simulink model "Reference_CVS"  (R2026a)
settings: Solver=ode1  StopTime=40
InitFcn:
  | %motor_control_init_m
  | %clear all
  | %close all
  | %clc
  | b=1e-8
  | StepSize = 1e-4;
  | N=1e-17;
  | 
  | VLV_0 =0;%120; %120
  | VA_0 = 0;%300; %300
  | VRV_0 = 0;%130;
  | VP_0 = 0;%500;
  | VLA_0 = 0;%20;
  | VV_0=5000;
  | VRA_0=0;
  | 
  | 
  | QLV_0 = 0;
  | QLA_0 = 0;
  | QP_0 = 0;
  | 
  | bh = 0;
  | th =0;
  | 
  | X_0 = [VLV_0 VA_0 VV_0 VP_0  VLA_0  VRA_0 VRV_0];
  | 
  | 
  | V0 = 10;
  | 
  | K1=.0004;%0.0001
  | K2=0.0009;%0.0009
  | KA=1;%1
  | C1=0.000000003;%0.0000003
  | lambda=6000;%3000
  | X_00 = [VLV_0 VA_0 VV_0 VRV_0];
  | 
  | r2 = 0.05/2;
  | A2 = pi*r2^2;
  | h2 = 0.63;
  | V2 = A2*h2;
  | 
  | 
  | r3 = 0.05/2;
  | A3 = pi*r3^2;
  | h3 = 0.63;
  | V3 = A3*h3;
  | 
  | 
  | rho = 997;
  | gg = 9.81;
  | %
  | init_min=0;
  | init_max=0;
  | %
  | PWM_Period =  StepSize;
  | PWM_Period_g1 = PWM_Period;
  | PWM_Period_g2 =PWM_Period;
  | PWM_Period_g3 = PWM_Period;
  | PWM_Period_g4 = PWM_Period;
  | PWM_Period_g5 = PWM_Period;
  | PWM_Period_P2_escape = PWM_Period;
  | PWM_Period_P3_escape = PWM_Period;
  | filter_c=100;
  | dt = StepSize;
  | dt_k = dt;
  | rho_g=1.537408456055604
  | Pvac = 0;
  | P1refmmHg = 1600;
  | P2refmmHg = 30;
  | 
  | 
  | P2_ref_freq = 1;
  | P2_ref_bias = 50;
  | P2_ref_amp = 0;
  | P2_ref_shift = 0;
  | Kp = 1;
  | Ki =1;
  | Kd=1;
  | 
  | 
  | P3_ref_freq = 1;
  | P3_ref_bias = 30;
  | P3_ref_amp = 0;
  | P3_ref_shift = 0;
  | 
  | Q_Sys_std = 1;
  | R_Meas_std = 1;
  | kalmanP_in= [133.32*[100 1 10 10 1]]';
  | kalmanQ_in = [1e-3 1e-3]';
  | y_kalman_ini = [133.32*[100 1 10 10 1] 1e-3 1e-3 1e-3]';
  | P_kalman_ini = R_Meas_std^2*eye(8);
  | %P_kalman_ini = R_Meas_std^2*eye(8);
  | %P_kalman_in1 = R_Meas_std^2*eye(8);
  | 
  | 
  | w_gp_0 = 1e-3;
  | i_gp_0 = 1e-3;
  | w_vad_0 = 1e-3;
  | i_vad_0 = 1e-3;
  | 
  | 
  | 
  | 
  | 
  | % e_min = 0.075;
  | % %e_max = 3;
  | % e_max_ill = 1.5; PA_0 = 85;
  | % tau_RA = 1.8;  tau_RV = 3;% 2.3762;
  | % V_total = 5500; V0_la = 70; V0_lv = 120; V0 = 10;
  | % RA = 1.2; Ra = 0.0005;
  | % Rm = 0.0003; Rv = 0.005;
  | % R = [RA Ra Rm Rv];
  | % g = [1/RA 1/Ra 1/Rm 1/Rv];
  | %
  | % CA = tau_RA/RA; CV = tau_RV/Rv;
  | %
  | % V0_aortic = PA_0*CA;
  | % PLV_0 = (V0_lv - V0)*e_min;
  | % CLA = V0_la/PLV_0;
  | % C = [CA CV CLA];
  | % e = [1/CA 1/CV 1/CLA];
  | %
  | % V0_venous = V_total - (V0_aortic + V0_la + V0_lv);
  | % PLA_0 = PLV_0;
  | % PV_0 = V0_venous/CV;
  | 
  | 
  | 
  | 
  | 
  | 
  | 
  | 
  | % stepsize = 1e-4;
  | 
  | % SS=1;
  | 
  | 
  | 
  | 
  | 
  | %global RFa RFp
  | %RFa = 1;
  | %RFmv = 1;
  | 
  | 
  | 
  | 
  | 
  | %L_AV =  0.000232;
  | %L_mv =  0.0001;
  | %L_P =  0.000128;
  | a=0;
  | 
  | 
  | 
  | 
  | 
  | %L= [L_mv];
  | 
  | 
  | 
  | 
  | 
  | % gLV =42;%25;
  | % gA = 0.9225;%0.75;  %0.8;%0.725; %1.11;
  | % gV = 70;%10000;
  | % gRV =210;
  | % gP =5;%15 %10;
  | % gLA = 1000; %1000;
  | %
  | %
  | % G = [gLV gA gV gRV gP gLA];
  | %
  | %
  | % eA =0.5225;%0.725;%1; %0.925;%0.83; %0.65;%0.95;
  | % eV =0.002425;%0.00245;%0.00125;
  | % eP =0.1; %0.01%0.1;
  | % eLA =0.1025;%0.1105%0.1175;%0.15; % 0.15;
  | %
  | %
  | % E = [eA eV eP eLA];
  | %
  | %
  | % ZZ = 0.75;
  | % PP = 0.95;
  | %
  | % V_T = 5000;
  | % VLV_0 =105;%120; %120
  | % VA_0 = 160;%300; %300
  | % VRV_0 = 110;%130;
  | % VP_0 = 200;%500;
  | % VLA_0 = 105;%20;
  | % VV_0=0;
  | % QLV_0 = 0;
  | % QLA_0 = 0;
  | % QP_0 = 0;
  | %
  | % X_0 = [VLV_0 VA_0 VRV_0 VP_0 VLA_0];
  | % %BF_0 = [0 0 0];
  | %
  | %
  | % V0 = 10;
  | 
  | 
  | %Delay = 0.85;
  | 
  | 
  | 
  | 
  | 
  | %%CVS PARAMETERS NEW
  | 
  | 
  | stepsize = 1e-4;
  | 
  | 
  | SS=0.8;
libraries: powerlib_meascontrol x12, simulink x8, cstblocks x6
(part 1 of 2)
settings Model: Creator=ehd  LastModifiedBy=ehd

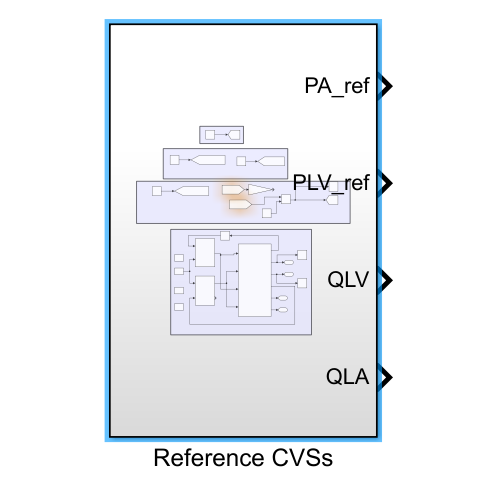
[thumbnail: Simulink's stored preview of the top-level diagram]
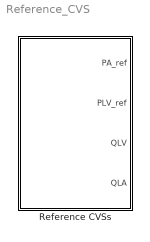
== system Reference_CVS ==
  Reference CVSs : Subsystem

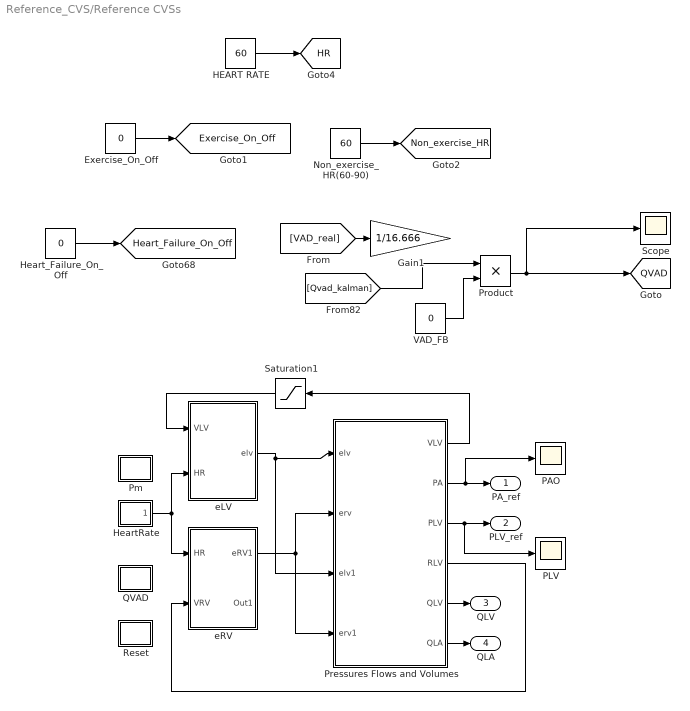
== system Reference_CVS/Reference CVSs ==
  Exercise_On_Off : Constant  Value=0
  Gain1 : Gain  Gain=1/16.666
  HEART RATE : Constant  Value=60
  HeartRate : Subsystem
  Heart_Failure_On_Off : Constant  Value=0
  Non_exercise_HR(60-90) : Constant  Value=60
  PAO : Scope
      settings: ActiveDisplayYMinimum=-0.039798343715390615  ActiveDisplayYMaximum=0.35818509343851557
  PLV : Scope
      settings: ActiveDisplayYMinimum=-23.924884385972419  ActiveDisplayYMaximum=6.1036636998176323  DataLoggingVariableName=ScopeData2
  Pm : Subsystem
  Pressures Flows and Volumes : Subsystem
  Product : Product
  QVAD : Subsystem
  Reset : Subsystem
  Saturation1 : Saturate  UpperLimit=500  LowerLimit=-100
  Scope : Scope
      settings: ActiveDisplayYMinimum=-1  ActiveDisplayYMaximum=1  DataLoggingVariableName=ScopeData3
  VAD_FB : Constant  Value=0
  eLV : Subsystem
  eRV : Subsystem
  PA_ref : Outport  VectorParamsAs1DForOutWhenUnconnected=off
  PLV_ref : Outport  Port=2  VectorParamsAs1DForOutWhenUnconnected=off
  QLV : Outport  Port=3  VectorParamsAs1DForOutWhenUnconnected=off
  QLA : Outport  Port=4  VectorParamsAs1DForOutWhenUnconnected=off
  tag scope: Exercise_On_Off=global, HR=global, Heart_Failure_On_Off=global, Non_exercise_HR=global, QVAD=global
  wires:
  Saturation1/1 -> eLV/1(VLV)
  [Qvad_kalman] -> Product/1
  [VAD_real] -> Gain1/1
  Pressures Flows and Volumes/5(QLV) -> QLV/1
  Pressures Flows and Volumes/6(QLA) -> QLA/1
  Pressures Flows and Volumes/2(PA) -> PA_ref/1, PAO/1
  Pressures Flows and Volumes/3(PLV) -> PLV_ref/1, PLV/1
  Pressures Flows and Volumes/1(VLV) -> Saturation1/1
  eLV/1(elv) -> Pressures Flows and Volumes/1(elv), Pressures Flows and Volumes/3(elv1)
  HeartRate/1(Out1) -> eLV/2(HR), eRV/1(HR)
  eRV/1(eRV1) -> Pressures Flows and Volumes/2(erv), Pressures Flows and Volumes/4(erv1)
  Pressures Flows and Volumes/4(RLV) -> eRV/2(VRV)
  VAD_FB/1 -> Product/2
  Product/1 -> [QVAD], Scope/1
  HEART RATE/1 -> [HR]
  Heart_Failure_On_Off/1 -> [Heart_Failure_On_Off]
  Non_exercise_HR(60-90)/1 -> [Non_exercise_HR]
  Exercise_On_Off/1 -> [Exercise_On_Off]

== system Reference_CVS/Reference CVSs/HeartRate ==
  Display : Display
  Display1 : Display
  Display2 : Display
  Switch2 : Switch  Criteria=u2 > Threshold  SaturateOnIntegerOverflow=off  InputSameDT=off
  Out1 : Outport
  tag scope: insan=global
  wires:
  Switch2/1 -> Display2/1, [insan]
  [Non_exercise_HR] -> Display1/1, Switch2/3
  [Exercise_On_Off] -> Switch2/2
  [HR] -> Display/1, Switch2/1, Out1/1

== system Reference_CVS/Reference CVSs/Pm ==
  note: y = -0,0333x 2 + 11,667x - 580
  note: y = -0,3333x2 + 116,67x - 5800R² = 1
  Add18 : Sum
  Add19 : Sum
  Constant20 : Constant  Value=-580
  Gain1 : Gain  Gain=1/100
  Gain2 : Gain  Gain=-0.0333
  Gain3 : Gain  Gain=11.667
  PID : Subsystem  Commented=on
  Product15 : Product
  Scope : Scope
      settings: ActiveDisplayYMinimum=3.007  ActiveDisplayYMaximum=5.007
  tag scope: PM=global
  wires:
  Gain1/1 -> Scope/1, [PM]
  Constant20/1 -> Add19/2
  Product15/1 -> Gain2/1
  Add18/1 -> Add19/1
  [HR] -> Gain3/1, Product15/2, Product15/1
  Gain3/1 -> Add18/2
  Gain2/1 -> Add18/1
  Add19/1 -> Gain1/1

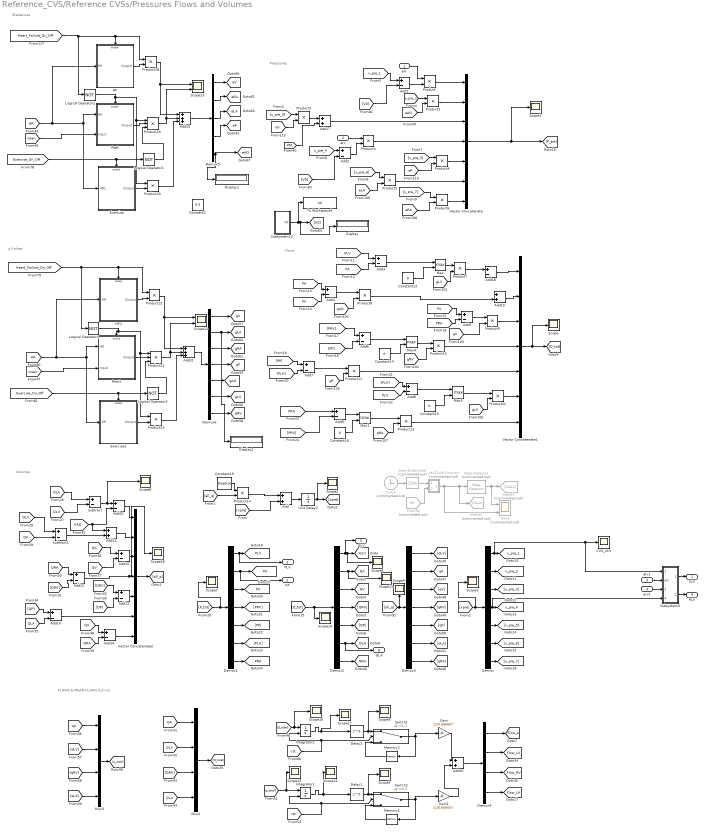
== system Reference_CVS/Reference CVSs/Pressures Flows and Volumes ==
  note: FLOWS & MEAN FLOWS (L/min)
  note: Elastances
  note: g Values
  note: Presssures
  note: Flows
  note: Volumes
  elv : Inport
  erv : Inport  Port=2
  elv1 : Inport  Port=3
  erv1 : Inport  Port=4
  Add{,11,17,19..20} (5 alike) : Sum
  Add{1..10,12..16,18} (16 alike) : Sum  Inputs=+-
  Add21 : Sum  Inputs=+++
  Add25 : Sum  Inputs=+++
  CVS_VLV : Scope
      settings: DataLoggingVariableName=ScopeData4
  Clock : Clock  Commented=on
      settings: Decimation=10000000
  Constant{13..16} (4 alike) : Constant  Value=0
  Constant19 : Constant  Value=stepsize
  Constant2 : Constant  Value=0.3
  Delay1 : Delay  DelayLength=5
  Delay2 : Delay  DelayLength=5
  Demux{,1..3,6} (5 alike) : Demux  Outputs=7
  Demux4 : Demux
  Demux5 : Demux  Outputs=5
  Display : Display
  Display1 : Display
  Display2 : Display
  Edge Detector : powerlib_meascontrol/Logic/Edge Detector  Commented=on  model=Falling  ic=0  Ts=0
      settings: SourceProductName=Simscape Electrical
  Exercise : Subsystem  TreatAsAtomicUnit=on
  Exercise2 : Subsystem  TreatAsAtomicUnit=on
  From90 : From  Commented=on  GotoTag=HR  TagVisibility=global
  Gain : Gain  Gain=1/16.666667
  Gain1 : Gain  Gain=1/16.666667
  Goto32 : Goto  Commented=on  GotoTag=Reset
  Goto55 : Goto  Commented=on  GotoTag=AAAA
  HF : Subsystem  TreatAsAtomicUnit=on
  HF1 : Subsystem  TreatAsAtomicUnit=on
  Integrator1 : Integrator  ExternalReset=either
  Integrator2 : Integrator  ExternalReset=either
  Logical Operator{1..4} (4 alike) : Logic  Operator=NOT  AllPortsSameDT=off  OutDataTypeStr=boolean
  MATLAB Function : MATLAB Function  Commented=on  TreatAsAtomicUnit=on
  Max{,1,4..5} (4 alike) : MinMax  Function=max  Inputs=2
  Memory1 : Memory  InheritSampleTime=on
  Memory2 : Memory  InheritSampleTime=on
  Mux2 : Mux
  Mux3 : Mux
  Product{,1..14,18,20..21,23} (19 alike) : Product
  Product19 : Product  Inputs=3
  Product22 : Product  Inputs=3
  Rest : Subsystem  TreatAsAtomicUnit=on
  Rest1 : Subsystem  TreatAsAtomicUnit=on
  Scope{,1..11,14..18} (17 alike) : Scope
      Scope settings: ActiveDisplayYMinimum=-77.48033  ActiveDisplayYMaximum=390.18057  DataLoggingVariableName=ScopeData3
      Scope1 settings: ActiveDisplayYMinimum=-17.90547  ActiveDisplayYMaximum=127.32097  DataLoggingVariableName=ScopeData4
      Scope10 settings: ActiveDisplayYMinimum=957.88839  ActiveDisplayYMaximum=957.93755  DataLoggingVariableName=ScopeData12
      Scope11 settings: ActiveDisplayYMinimum=-27.48687  ActiveDisplayYMaximum=51.0539  DataLoggingVariableName=ScopeData10
      Scope14 settings: ActiveDisplayYMinimum=-110.80263  ActiveDisplayYMaximum=77.31742
      Scope15 settings: ActiveDisplayYMinimum=-5789.58317  ActiveDisplayYMaximum=-2381.5007  DataLoggingVariableName=ScopeData2
      Scope16 settings: ActiveDisplayYMinimum=1027.76879  ActiveDisplayYMaximum=5015.29115  DataLoggingVariableName=ScopeData3
      Scope17 settings: ActiveDisplayYMinimum=-44.98014  ActiveDisplayYMaximum=404.82124  DataLoggingVariableName=ScopeData4
      Scope18 settings: ActiveDisplayYMinimum=2390.88881  ActiveDisplayYMaximum=2481.24108  DataLoggingVariableName=ScopeData5
      Scope2 settings: ActiveDisplayYMinimum=-34.04375  ActiveDisplayYMaximum=306.39376  DataLoggingVariableName=ScopeData3
      Scope3 settings: ActiveDisplayYMinimum=-92.27651  ActiveDisplayYMaximum=239.55796  DataLoggingVariableName=ScopeData3
      Scope4 settings: ActiveDisplayYMinimum=-3614.79854  ActiveDisplayYMaximum=3696.63533
      Scope5 settings: ActiveDisplayYMinimum=-10.26706  ActiveDisplayYMaximum=83.80402  DataLoggingVariableName=ScopeData2
      Scope6 settings: ActiveDisplayYMinimum=-1637.52208  ActiveDisplayYMaximum=5158.92158  DataLoggingVariableName=ScopeData9
      Scope7 settings: ActiveDisplayYMinimum=75.32296  ActiveDisplayYMaximum=84.1275  DataLoggingVariableName=ScopeData3
      Scope8 settings: ActiveDisplayYMinimum=-106.50454  ActiveDisplayYMaximum=958.54088  DataLoggingVariableName=ScopeData10
      Scope9 settings: ActiveDisplayYMinimum=-10.26706  ActiveDisplayYMaximum=83.80402  DataLoggingVariableName=ScopeData3
  Scope12 : Scope  NumInputPorts=2
      settings: ActiveDisplayYMinimum=-0.0275  ActiveDisplayYMaximum=0.2475  DataLoggingVariableName=ScopeData3
  Scope13 : Scope  NumInputPorts=2
      settings: ActiveDisplayYMinimum=-31.25  ActiveDisplayYMaximum=281.25  DataLoggingVariableName=ScopeData2
  Subsystem13 : Subsystem
  Subsystem5 : Subsystem
  Subtract : Sum  Inputs=+-
  Subtract1 : Sum  Inputs=+-
  Switch1 : Switch  Threshold=1  SaturateOnIntegerOverflow=off  InputSameDT=off
  Switch2 : Switch  Threshold=1  SaturateOnIntegerOverflow=off  InputSameDT=off
  To Workspace5 : ToWorkspace  VariableName=V0  SampleTime=-1
      settings: Save2DSignal=2-D array (concatenate along first dimension)
  Unit Delay2 : UnitDelay  InitialCondition=X_0  SampleTime=-1
  Vector Concatenate : Concatenate  NumInputs=7
  Vector Concatenate1 : Concatenate  NumInputs=7
  Vector Concatenate2 : Concatenate  NumInputs=7
  Wave : Scope  Commented=on  NumInputPorts=2
      settings: ActiveDisplayYMinimum=-0.125  ActiveDisplayYMaximum=1.125  DataLoggingVariableName=ScopeData2
  Zero-Order Hold : ZeroOrderHold  Commented=on  SampleTime=-1
  VLV : Outport
  PA : Outport  Port=2  VectorParamsAs1DForOutWhenUnconnected=off
  PLV : Outport  Port=3  VectorParamsAs1DForOutWhenUnconnected=off
  RLV : Outport  Port=4
  QLV : Outport  Port=5  VectorParamsAs1DForOutWhenUnconnected=off
  QLA : Outport  Port=6  VectorParamsAs1DForOutWhenUnconnected=off
  tag scope: Flow_A=global, Flow_LA=global, Flow_LV=global, Flow_RV=global, PA=global, PLV=global, PRA=global, PV=global, QA=global, QLA=global, QLV=global, QRA=global, QV=global, eAO=global, eLA=global, eP=global, eRA=global, eV=global, gAO=global, gLA=global, gLV=global, gP=global, gRA=global, gRV=global, gV=global, qA=global, x_pre_1=global, x_pre_2=global, x_pre_4=global
  wires:
  Product12/1 -> Vector Concatenate1/6
  [QRV] -> Mux2/3
  [QA] -> Mux2/1
  Mux2/1 -> [Q_total]
  Demux4/1 -> [Flow_A]
  [qLV] -> Mux3/2
  Mux3/1 -> [q_total]
  [qRV] -> Mux3/3
  [qA] -> Mux3/1
  [QLV] -> Mux2/2
  [qLA] -> Mux3/4
  Add20/1 -> Demux4/1
  Demux4/4 -> [Flow_LA]
  Switch1/1 -> Gain/1, Memory2/1
  [QLA] -> Mux2/4
  Gain1/1 -> Add20/2
  Integrator2/1 -> Delay2/1, Scope17/1
  Memory2/1 -> Switch1/3
  [q_total] -> Integrator1/1, Scope15/1
  Integrator1/1 -> Delay1/1, Scope14/1
  Demux4/2 -> [Flow_LV]
  Memory1/1 -> Switch2/3
  Demux4/3 -> [Flow_RV]
  Delay2/1 -> Switch1/1, Scope9/1
  [Q_total] -> Integrator2/1, Scope16/1
  Delay1/1 -> Scope5/1, Switch2/1
  Switch2/1 -> Memory1/1, Gain1/1
  [rst] -> Switch2/2, Integrator1/2
  Gain/1 -> Add20/1
  [rst] -> Integrator2/2, Switch1/2
  Demux2/2 -> [QA], Scope11/1
  Demux5/5 -> Display1/1, [eAO]
  Demux6/5 -> [gAO]
  Product1/1 -> Vector Concatenate/2
  [eAO] -> Product1/2
  [x_pre_2] -> Product1/1
  Subsystem13/1(V0) -> [V0], Display/1, To Workspace5/1
  [HR] -> Rest1/1(HR), Exercise2/1(HR), HF1/1(HR)
  Demux5/3 -> [eLA]
  [Exercise_On_Off] -> Exercise/Enable, Logical Operator1/1
  Product19/1 -> Add25/2, Scope13/2
  Product21/1 -> Scope12/1, Add21/1
  Logical Operator1/1 -> Product19/3
  Demux6/7 -> [gRV]
  Logical Operator2/1 -> Rest/Enable, Product19/1, Product20/1
  Rest/1(Output) -> Product19/2
  [Exercise_On_Off] -> Exercise2/Enable, Logical Operator3/1
  Add25/1 -> Demux5/1
  [HR] -> Rest/1(HR), Exercise/1(HR1), HF/1(HR)
  Demux6/6 -> [gLV]
  Add21/1 -> Demux6/1
  Logical Operator4/1 -> Product22/1, Product23/1, Rest1/Enable
  HF1/1(Output) -> Product21/2
  Demux6/2 -> [gLA], Display2/1
  Demux6/1 -> [gV]
  [Heart_Failure_On_Off] -> HF/Enable, Product18/1, Logical Operator2/1
  [insan] -> Rest/2(Input)
  Demux5/4 -> [eP]
  Demux6/4 -> [gP]
  Product22/1 -> Add21/2, Scope12/2
  Product18/1 -> Scope13/1, Add25/1
  Exercise/1(Output) -> Product20/2
  Product20/1 -> Add25/3
  Logical Operator3/1 -> Product22/3
  Product23/1 -> Add21/3
  [Heart_Failure_On_Off] -> Logical Operator4/1, Product21/1, HF1/Enable
  Exercise2/1(Output) -> Product23/2
  Demux5/1 -> [eV]
  Rest1/1(Output) -> Product22/2
  Demux6/3 -> [gRA]
  Demux5/2 -> [eRA]
  HF/1(Output) -> Product18/2
  [insan] -> Rest1/2(Input)
  Demux/1 -> [x_pre_1], CVS_VLV/1, Subsystem5/1(In1)
  elv1/1 -> Subsystem5/2(elv)
  erv1/1 -> Subsystem5/3(erv)
  Demux/4 -> [x_pre_4], Subsystem5/4(In4)
  Subsystem5/1(Out1) -> VLV/1
  Subsystem5/2(Output1) -> RLV/1
  [PM] -> Add17/2
  [VAD] -> Add10/2, Add11/1
  Demux2/4 -> [QRV]
  [all_q] -> Scope4/1, Demux3/1
  Demux/2 -> [x_pre_2]
  From90/1 -> MATLAB Function/2(HR)
  MATLAB Function/1(y) -> Goto32/1, Edge Detector/1, Wave/2
  Demux1/2 -> [PA], PA/1
  Add19/1 -> Vector Concatenate1/2
  Product8/1 -> Add19/2
  Add18/1 -> Vector Concatenate1/1
  Product7/1 -> Add18/1
  Add11/1 -> Vector Concatenate2/2
  Add10/1 -> Vector Concatenate2/1
  Subtract1/1 -> Add11/2
  Subtract/1 -> Add10/1, Scope6/1
  [eV] -> Product2/2
  [V0] -> Add2/2
  [V0] -> Add1/2
  [eP] -> Product4/2
  [eLA] -> Product5/2
  [eRA] -> Product6/2
  [gRA] -> Product13/2
  [gLA] -> Product12/2
  [gP] -> Product11/2
  [gRV] -> Product10/2
  [gV] -> Product9/2
  [gAO] -> Product8/2
  [gLV] -> Product7/2
  Edge Detector/1 -> Goto55/1, Wave/1
  Demux3/7 -> [qRA]
  Demux3/6 -> [qLA]
  Demux3/5 -> [qP]
  Demux3/4 -> [qRV]
  Demux3/3 -> [qV]
  Demux3/2 -> [qA]
  Demux3/1 -> [qLV]
  Zero-Order Hold/1 -> MATLAB Function/1(u)
  Clock/1 -> Zero-Order Hold/1
  [QLV] -> Subtract/2
  Product9/1 -> Vector Concatenate1/3
  [Q_tot] -> Demux2/1, Scope10/1
  Unit Delay2/1 -> [xpre], Scope2/1
  Add/1 -> Unit Delay2/1
  Constant19/1 -> Product14/1
  Add14/1 -> Vector Concatenate2/6
  Add13/1 -> Vector Concatenate2/5
  Add12/1 -> Vector Concatenate2/4, Scope18/1
  Add15/1 -> Vector Concatenate2/3
  [x_pre_7] -> Product6/1
  [x_pre_6] -> Product5/1
  [x_pre_5] -> Product4/1
  [x_pre_4] -> Add2/1
  [x_pre_3] -> Product2/1
  Constant13/1 -> Max/2
  Add3/1 -> Max/1
  Add6/1 -> Max4/1
  Add9/1 -> Max1/1
  Add8/1 -> Max5/1
  Add17/1 -> Vector Concatenate/3
  Product2/1 -> Add17/1
  [all_q] -> Product14/2
  Vector Concatenate2/1 -> [all_q]
  Vector Concatenate1/1 -> Scope/1, [Q_tot]
  Vector Concatenate/1 -> Scope1/1, [P_tot]
  [QRA] -> Add16/2
  [QV] -> Add16/1
  Add16/1 -> Vector Concatenate2/7
  [QV] -> Add15/2
  [QA] -> Add15/1
  [QLA] -> Add14/2
  [QP] -> Add14/1
  [QP] -> Add13/2
  [QRV] -> Add13/1
  [QRV] -> Add12/2
  [QRA] -> Add12/1
  [QA] -> Subtract1/2
  [QLV] -> Subtract1/1
  [QLA] -> Subtract/1
  Demux2/3 -> [QV]
  Demux2/6 -> [QLA], QLA/1
  Demux2/5 -> [QP]
  Demux2/7 -> [QRA]
  Demux2/1 -> [QLV], Scope8/1, QLV/1
  Product13/1 -> Vector Concatenate1/7
  Max1/1 -> Product13/1
  Constant16/1 -> Max1/2
  [PRV] -> Add9/2
  [PRA] -> Add9/1
  Max5/1 -> Product12/1
  Constant15/1 -> Max5/2
  [PLV] -> Add8/2
  [PLA] -> Add8/1
  Product11/1 -> Vector Concatenate1/5
  Add7/1 -> Product11/1
  [PLA] -> Add7/2
  [PP] -> Add7/1
  Product10/1 -> Vector Concatenate1/4
  Max4/1 -> Product10/1
  [PP] -> Add6/2
  [PRV] -> Add6/1
  Constant14/1 -> Max4/2
  Add5/1 -> Product9/1
  [PRA] -> Add5/2
  [PV] -> Add5/1
  Add4/1 -> Product8/1
  [PV] -> Add4/2
  [PA] -> Add4/1
  Max/1 -> Product7/1
  [PA] -> Add3/2
  [PLV] -> Add3/1
  Demux1/3 -> [PV]
  Demux1/4 -> [PRV]
  Demux1/5 -> [PP]
  Demux1/6 -> [PLA]
  Demux1/7 -> [PRA]
  Demux1/1 -> [PLV], PLV/1
  [P_tot] -> Demux1/1, Scope7/1
  Product6/1 -> Vector Concatenate/7
  Product5/1 -> Vector Concatenate/6
  Product4/1 -> Vector Concatenate/5
  erv/1 -> Product3/1
  Product3/1 -> Vector Concatenate/4
  Add2/1 -> Product3/2
  Product/1 -> Vector Concatenate/1
  Add1/1 -> Product/2
  [x_pre_1] -> Add1/1
  Demux/7 -> [x_pre_7]
  Demux/6 -> [x_pre_6]
  Demux/5 -> [x_pre_5]
  Demux/3 -> [x_pre_3]
  [xpre] -> Demux/1, Scope3/1
  elv/1 -> Product/1
  [xpre] -> Add/2
  Product14/1 -> Add/1

== system Reference_CVS/Reference CVSs/QVAD ==
  Gain3 : Gain  Gain=16.666
  Product : Product
  Saturation : Saturate  UpperLimit=inf  LowerLimit=30
  Sine Wave : Sin  Amplitude=0.8  Frequency=0.4  SampleTime=0
  tag scope: VAD=global, VADQ=global
  wires:
  [QVAD] -> Gain3/1, [VADQ]
  Product/1 -> Saturation/1
  Sine Wave/1 -> Product/2
  Gain3/1 -> Product/1, [VAD]

== system Reference_CVS/Reference CVSs/Reset ==
  Clock2 : Clock
  Constant10 : Constant
  Constant11 : Constant  Value=0
  Constant12 : Constant  Value=10
  Mod2 : Math  Operator=mod  SignedPower=on
  Scope5 : Scope
      settings: ActiveDisplayYMinimum=-0.125  ActiveDisplayYMaximum=1.125  DataLoggingVariableName=ScopeData4
  Switch2 : Switch  Threshold=10-000001  SaturateOnIntegerOverflow=off  InputSameDT=off
  tag scope: dedect=global, rst=global
  wires:
  Clock2/1 -> Mod2/1
  Constant12/1 -> Mod2/2
  Constant10/1 -> Switch2/1
  Switch2/1 -> [rst], Scope5/1
  Constant11/1 -> Switch2/3
  Mod2/1 -> [dedect], Switch2/2

== system Reference_CVS/Reference CVSs/eLV ==
  VLV : Inport
  HR : Inport  Port=2
  Clock1 : Clock
  Constant : Constant  Value=3
  Display : Display
  LV_e_min : Subsystem
  Scope : Scope
      settings: ActiveDisplayYMinimum=-0.72024  ActiveDisplayYMaximum=3.41705
  Subsystem1 : Subsystem
  Switch : Switch  Criteria=u2 > Threshold  Threshold=0.9  SaturateOnIntegerOverflow=off  InputSameDT=off
  Switch1 : Switch  Criteria=u2 > Threshold  Threshold=0.9  SaturateOnIntegerOverflow=off  InputSameDT=off
  eLV1 : Subsystem
  eLVsick : Subsystem
  elv : Outport
  tag scope: eLV=global
  wires:
  eLVsick/1(Output) -> Switch/1
  Switch/1 -> Subsystem1/1(eLV_max), Display/1
  eLV1/1(Output) -> Switch1/1
  [Exercise_On_Off] -> Switch1/2
  Constant/1 -> Switch1/3
  Switch1/1 -> Switch/3
  [Heart_Failure_On_Off] -> Switch/2
  LV_e_min/1(eLV_min_O) -> Subsystem1/2(eLV_min)
  HR/1 -> Subsystem1/3(HR)
  VLV/1 -> LV_e_min/1(VLV)
  Subsystem1/1(elv) -> elv/1, [eLV], Scope/1
  Clock1/1 -> Subsystem1/4(t)

== system Reference_CVS/Reference CVSs/eRV ==
  HR : Inport
  VRV : Inport  Port=2
  Clock2 : Clock
  Display : Display
  RV_e_min : Subsystem
  Subsystem2 : Subsystem
  Switch : Switch  Criteria=u2 > Threshold  Threshold=0.9  SaturateOnIntegerOverflow=off  InputSameDT=off
  eRV2 : Subsystem
  eRVhf : Subsystem
  eRV1 : Outport
  Out1 : Outport  Port=2
  tag scope: eRV=global
  wires:
  Switch/1 -> Subsystem2/1(eRV_max), Display/1
  [Heart_Failure_On_Off] -> Switch/2
  eRVhf/1(Output) -> Switch/1
  eRV2/1(Output) -> Switch/3
  RV_e_min/1(eRV_min_O) -> Subsystem2/2(eRV_min)
  Subsystem2/1(eRV) -> eRV1/1, [eRV], Out1/1
  VRV/1 -> RV_e_min/1(VRV)
  HR/1 -> Subsystem2/4(HR)
  Clock2/1 -> Subsystem2/3(t)

== system Reference_CVS/Reference CVSs/Pm/PID ==
  s : Inport
  LTI System : cstblocks/LTI System  sys=tfa  IC=[]
  PID Controller : simulink/Continuous/PID Controller  Controller=PID  Form=Parallel  TimeDomain=Continuous-time  SampleTime=-1  IntegratorMethod=Forward Euler  FilterMethod=Forward Euler  ControllerParametersSource=internal  P=0  I=0.336541519886425  D=0  UseFilter=on  N=100  TunerSelectOption=Transfer Function Based (PID Tuner App)  InitialConditionSource=internal  InitialConditionForIntegrator=0  InitialConditionForFilter=0  DifferentiatorICPrevScaledInput=0  ExternalReset=none  TrackingMode=off  Kt=1  LimitOutput=off  UpperSaturationLimit=inf  LowerSaturationLimit=-inf  LinearizeAsGain=on  AntiWindupMode=none  Kb=1  POutMin=[]  POutMax=[]  IOutMin=[]  IOutMax=[]  DOutMin=[]  DOutMax=[]  NOutMin=[]  NOutMax=[]  SumOutMin=[]  SumOutMax=[]  SaturationOutMin=[]  SaturationOutMax=[]  PParamMin=[]  PParamMax=[]  IParamMin=[]  IParamMax=[]  DParamMin=[]  DParamMax=[]  NParamMin=[]  NParamMax=[]  KbParamMin=[]  KbParamMax=[]  KtParamMin=[]  KtParamMax=[]  KbOutMin=[]  KbOutMax=[]  KtOutMin=[]  KtOutMax=[]  IntegratorOutMin=[]  IntegratorOutMax=[]  FilterOutMin=[]  FilterOutMax=[]  SumI1OutMin=[]  SumI1OutMax=[]  SumI2OutMin=[]  SumI2OutMax=[]  SumI3OutMin=[]  SumI3OutMax=[]  SumI4OutMin=[]  SumI4OutMax=[]  SumDOutMin=[]  SumDOutMax=[]  DifferentiatorOutMin=[]  DifferentiatorOutMax=[]  FilterDiffOutCoefMin=[]  FilterDiffOutCoefMax=[]  ReciprocalOutMin=[]  ReciprocalOutMax=[]  SumDenOutMin=[]  SumDenOutMax=[]  SumNumOutMin=[]  SumNumOutMax=[]  DivideOutMin=[]  DivideOutMax=[]  IntegratorContinuousStateAttributes=''  IntegratorStateMustResolveToSignalObject=off  IntegratorRTWStateStorageClass=Auto  FilterContinuousStateAttributes=''  FilterStateMustResolveToSignalObject=off  FilterRTWStateStorageClass=Auto  ParallelPVariant=InternalParameters  IdealPVariant=Disabled  IVariant=InternalParameters  DVariant=InternalParameters  IntegratorVariant=Continuous  SatVariant=Disabled  AWVariant=Passthrough  PCopyVariant=Disabled  TRVariant=Disabled  FdbkBlocksVariant=Forward  IdealPFdbkVariant=Disabled  SatFdbkVariant=Disabled  DerivativeFilterVariant=ContFilter  NVariant=InternalParameters  NCopyVariant=Disabled  FilterICVariant=InternalICsFilter  IntegratorICVariant=InternalICs  ExternalResetVariant=Disabled  TRSumVariant=Passthrough  SumFdbkVariant=Disabled  SumVariant=Sum_PID
  Sum1 : Sum  Inputs=|+-
  To Workspace : ToWorkspace  VariableName=input  SampleTime=-1
  To Workspace1 : ToWorkspace  VariableName=output  SampleTime=-1
  E : Outport  VectorParamsAs1DForOutWhenUnconnected=off
  wires:
  PID Controller/1 -> To Workspace/1, LTI System/1
  s/1 -> Sum1/1
  Sum1/1 -> PID Controller/1
  LTI System/1 -> Sum1/2, E/1, To Workspace1/1

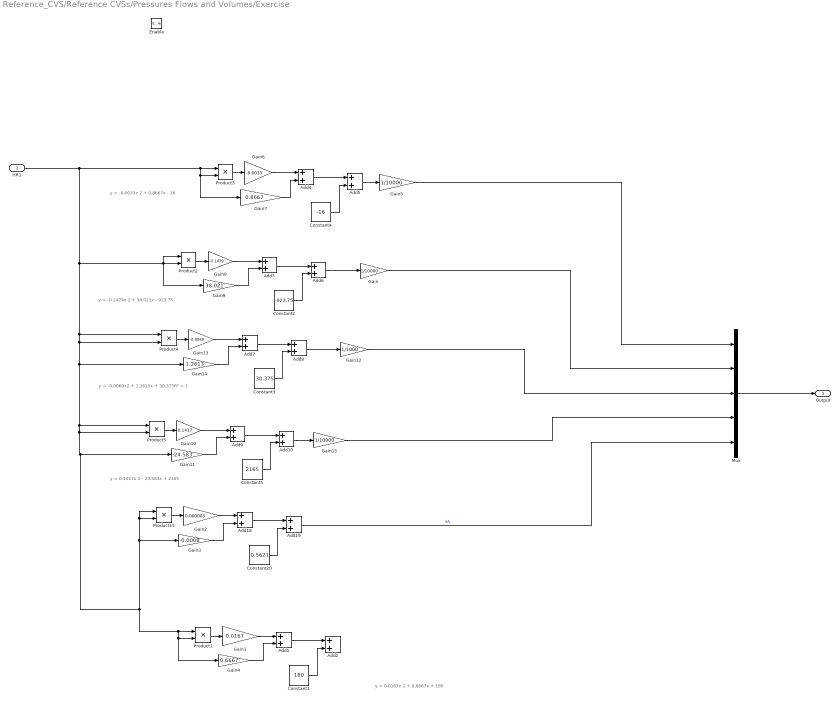
== system Reference_CVS/Reference CVSs/Pressures Flows and Volumes/Exercise ==
  note: y = -0,0033x 2 + 0,8667x - 16
  note: y = 0,1417x 2 - 24,583x + 2165
  note: y = -0,1479x 2 + 38,021x - 923,75
  note: y = -0,0069x2 + 1,2813x + 30,375R² = 1
  note: y = 0,0167x 2 + 0,6667x + 180
  HR1 : Inport
  Enable : EnablePort
  Add{1..10,18..19} (12 alike) : Sum
  Constant1 : Constant  Value=180
  Constant2 : Constant  Value=-923.75
  Constant20 : Constant  Value=0.5621
  Constant3 : Constant  Value=30.375
  Constant4 : Constant  Value=-16
  Constant5 : Constant  Value=2165
  Gain : Gain  Gain=1/10000
  Gain1 : Gain  Gain=0.0167
  Gain10 : Gain  Gain=0.1417
  Gain11 : Gain  Gain=-24.583
  Gain12 : Gain  Gain=1/1000
  Gain13 : Gain  Gain=-0.0069
  Gain14 : Gain  Gain=1.2813
  Gain15 : Gain  Gain=1/10000
  Gain2 : Gain  Gain=0.000003
  Gain3 : Gain  Gain=-0.0008
  Gain4 : Gain  Gain=0.6667
  Gain5 : Gain  Gain=1/10000
  Gain6 : Gain  Gain=-0.0033
  Gain7 : Gain  Gain=0.8667
  Gain8 : Gain  Gain=-0.1479
  Gain9 : Gain  Gain=38.021
  Mux : Mux  Inputs=5
  Product{1..5,15} (6 alike) : Product
  Output : Outport
  wires:
  Gain15/1 -> Mux/4
  Gain/1 -> Mux/2
  Product5/1 -> Gain10/1
  Gain7/1 -> Add4/2
  Gain14/1 -> Add7/2
  Product3/1 -> Gain6/1
  Gain5/1 -> Mux/1
  Add7/1 -> Add8/1
  Product2/1 -> Gain8/1
  Add5/1 -> Gain5/1
  Add6/1 -> Gain/1
  Constant2/1 -> Add6/2
  Gain6/1 -> Add4/1
  Add4/1 -> Add5/1
  Constant4/1 -> Add5/2
  Gain13/1 -> Add7/1
  Constant3/1 -> Add8/2
  Add10/1 -> Gain15/1
  Gain12/1 -> Mux/3
  Add8/1 -> Gain12/1
  Product4/1 -> Gain13/1
  Gain8/1 -> Add3/1
  Gain9/1 -> Add3/2
  Add3/1 -> Add6/1
  Add9/1 -> Add10/1
  Gain11/1 -> Add9/2
  Constant5/1 -> Add10/2
  Gain10/1 -> Add9/1
  Mux/1 -> Output/1
  Gain4/1 -> Add1/2
  Gain1/1 -> Add1/1
  Product1/1 -> Gain1/1
  Add1/1 -> Add2/1
  HR1/1 -> Product3/1, Product3/2, Gain7/1, Gain11/1, Product1/1, Product1/2, Gain4/1, Gain3/1, Product15/2, Product15/1, Product5/2, Product5/1, Gain14/1, Product4/2, Product4/1, Product2/2, Gain9/1, Product2/1
  Constant1/1 -> Add2/2
  Gain2/1 -> Add18/1
  Gain3/1 -> Add18/2
  Add18/1 -> Add19/1
  Constant20/1 -> Add19/2
  Product15/1 -> Gain2/1
  Add19/1 -> Mux/5  "eA"

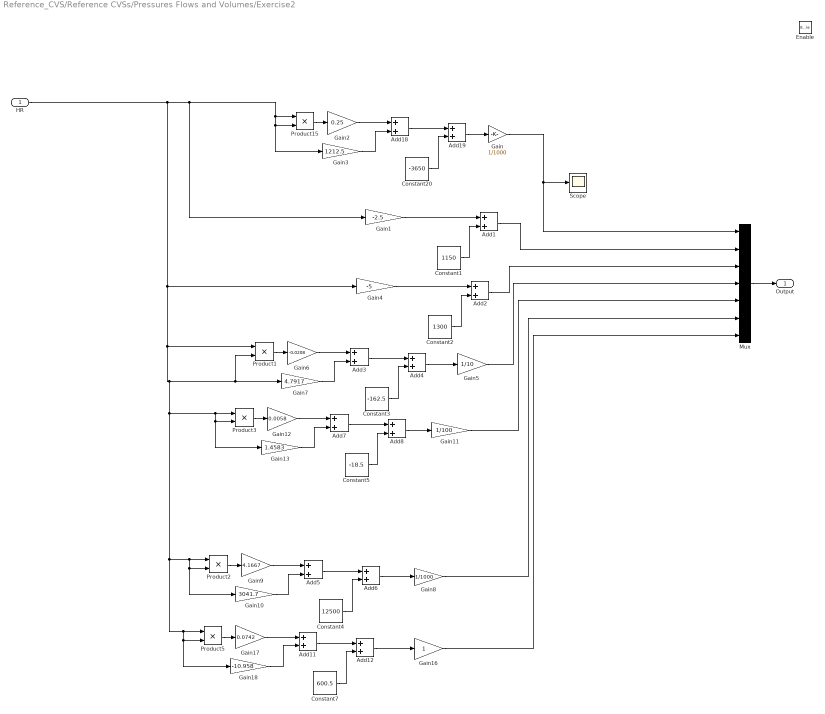
== system Reference_CVS/Reference CVSs/Pressures Flows and Volumes/Exercise2 ==
  HR : Inport
  Enable : EnablePort
  Add{1..8,11..12,18..19} (12 alike) : Sum
  Constant1 : Constant  Value=1150
  Constant2 : Constant  Value=1300
  Constant20 : Constant  Value=-3650
  Constant3 : Constant  Value=-162.5
  Constant4 : Constant  Value=12500
  Constant5 : Constant  Value=-18.5
  Constant7 : Constant  Value=600.5
  Gain : Gain  Gain=1/1000
  Gain1 : Gain  Gain=-2.5
  Gain10 : Gain  Gain=3041.7
  Gain11 : Gain  Gain=1/100
  Gain12 : Gain  Gain=0.0058
  Gain13 : Gain  Gain=1.4583
  Gain16 : Gain
  Gain17 : Gain  Gain=0.0742
  Gain18 : Gain  Gain=-10.958
  Gain2 : Gain  Gain=0.25
  Gain3 : Gain  Gain=1212.5
  Gain4 : Gain  Gain=-5
  Gain5 : Gain  Gain=1/10
  Gain6 : Gain  Gain=-0.0208
  Gain7 : Gain  Gain=4.7917
  Gain8 : Gain  Gain=1/1000
  Gain9 : Gain  Gain=4.1667
  Mux : Mux  Inputs=7
  Product{1..3,5,15} (5 alike) : Product
  Scope : Scope
      settings: ActiveDisplayYMinimum=60  ActiveDisplayYMaximum=80  DataLoggingVariableName=ScopeData9
  Output : Outport
  wires:
  Gain18/1 -> Add11/2
  Gain16/1 -> Mux/7
  Gain17/1 -> Add11/1
  HR/1 -> Gain4/1, Product1/1, Product3/1, Product3/2, Gain13/1, Gain18/1, Product5/2, Product5/1, Product2/1, Product2/2, Gain10/1, Product1/2, Gain7/1, Gain1/1, Product15/1, Product15/2, Gain3/1
  Add12/1 -> Gain16/1
  Constant7/1 -> Add12/2
  Add11/1 -> Add12/1
  Product5/1 -> Gain17/1
  Gain13/1 -> Add7/2
  Gain11/1 -> Mux/5
  Add8/1 -> Gain11/1
  Product3/1 -> Gain12/1
  Constant5/1 -> Add8/2
  Add7/1 -> Add8/1
  Gain12/1 -> Add7/1
  Mux/1 -> Output/1
  Gain2/1 -> Add18/1
  Gain/1 -> Mux/1, Scope/1
  Constant20/1 -> Add19/2
  Product15/1 -> Gain2/1
  Gain3/1 -> Add18/2
  Add19/1 -> Gain/1
  Add18/1 -> Add19/1
  Add1/1 -> Mux/2
  Constant1/1 -> Add1/2
  Gain1/1 -> Add1/1
  Gain4/1 -> Add2/1
  Add2/1 -> Mux/3
  Constant2/1 -> Add2/2
  Constant3/1 -> Add4/2
  Gain7/1 -> Add3/2
  Gain5/1 -> Mux/4
  Product1/1 -> Gain6/1
  Gain6/1 -> Add3/1
  Add4/1 -> Gain5/1
  Add3/1 -> Add4/1
  Add6/1 -> Gain8/1
  Constant4/1 -> Add6/2
  Gain10/1 -> Add5/2
  Gain8/1 -> Mux/6
  Add5/1 -> Add6/1
  Product2/1 -> Gain9/1
  Gain9/1 -> Add5/1

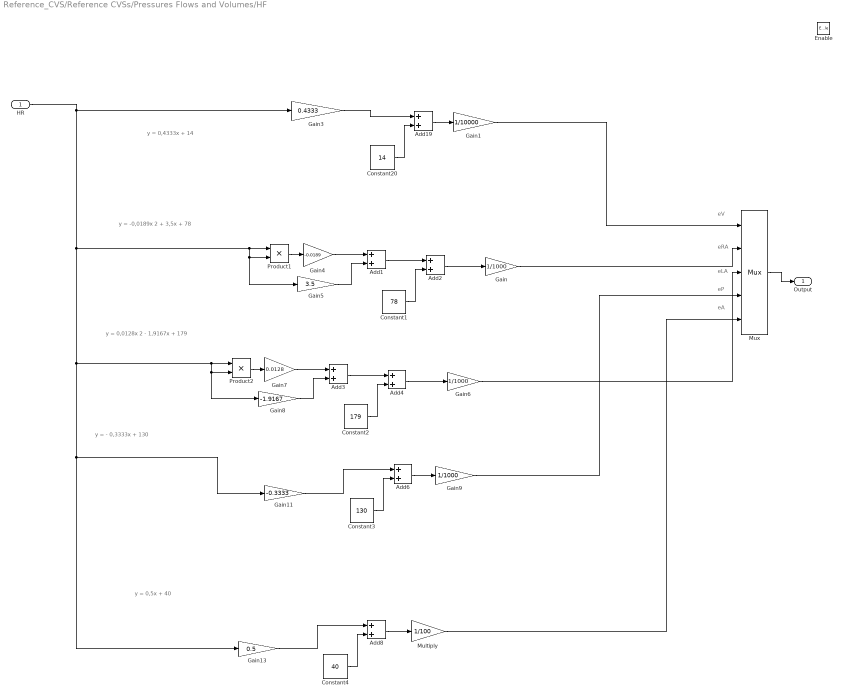
== system Reference_CVS/Reference CVSs/Pressures Flows and Volumes/HF ==
  note: eA
  note: eP
  note: eLA
  note: eRA
  note: eV
  note: y = 0,4333x + 14
  note: y = -0,0189x 2 + 3,5x + 78
  note: y = 0,0128x 2 - 1,9167x + 179
  note: y = - 0,3333x + 130
  note: y = 0,5x + 40
  HR : Inport
  Enable : EnablePort
  Add{1..4,6,8,19} (7 alike) : Sum
  Constant1 : Constant  Value=78
  Constant2 : Constant  Value=179
  Constant20 : Constant  Value=14
  Constant3 : Constant  Value=130
  Constant4 : Constant  Value=40
  Gain : Gain  Gain=1/1000
  Gain1 : Gain  Gain=1/10000
  Gain11 : Gain  Gain=-0.3333
  Gain13 : Gain  Gain=0.5
  Gain3 : Gain  Gain=0.4333
  Gain4 : Gain  Gain=-0.0189
  Gain5 : Gain  Gain=3.5
  Gain6 : Gain  Gain=1/1000
  Gain7 : Gain  Gain=0.0128
  Gain8 : Gain  Gain=-1.9167
  Gain9 : Gain  Gain=1/1000
  Multiply : Gain  Gain=1/100
  Mux : Mux  Inputs=5
  Product1 : Product
  Product2 : Product
  Output : Outport
  wires:
  HR/1 -> Gain3/1, Gain8/1, Product2/2, Product2/1, Gain11/1, Gain13/1, Gain5/1, Product1/2, Product1/1
  Gain13/1 -> Add8/1
  Constant4/1 -> Add8/2
  Add8/1 -> Multiply/1
  Multiply/1 -> Mux/5
  Mux/1 -> Output/1
  Gain9/1 -> Mux/4
  Constant3/1 -> Add6/2
  Gain11/1 -> Add6/1
  Add6/1 -> Gain9/1
  Gain6/1 -> Mux/3
  Product2/1 -> Gain7/1
  Constant2/1 -> Add4/2
  Add4/1 -> Gain6/1
  Gain8/1 -> Add3/2
  Gain7/1 -> Add3/1
  Add3/1 -> Add4/1
  Constant1/1 -> Add2/2
  Gain5/1 -> Add1/2
  Add2/1 -> Gain/1
  Gain4/1 -> Add1/1
  Product1/1 -> Gain4/1
  Gain/1 -> Mux/2
  Add1/1 -> Add2/1
  Add19/1 -> Gain1/1
  Gain1/1 -> Mux/1
  Constant20/1 -> Add19/2
  Gain3/1 -> Add19/1

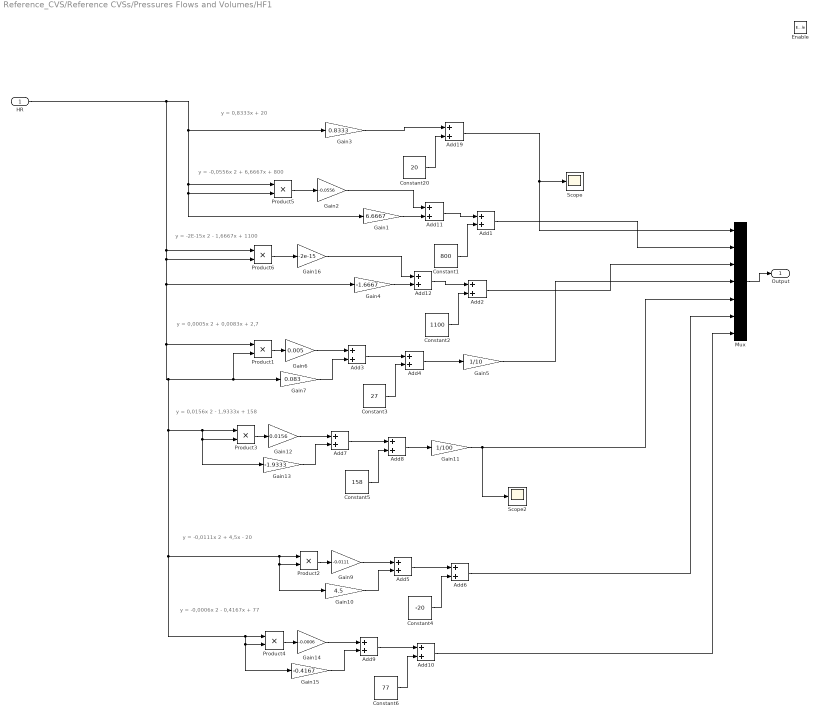
== system Reference_CVS/Reference CVSs/Pressures Flows and Volumes/HF1 ==
  note: y = -0,0006x 2 - 0,4167x + 77
  note: y = 0,0156x 2 - 1,9333x + 158
  note: y = -0,0556x 2 + 6,6667x + 800
  note: y = 0,0005x 2 + 0,0083x + 2,7
  note: y = 0,8333x + 20
  note: y = -2E-15x 2 - 1,6667x + 1100
  note: y = -0,0111x 2 + 4,5x - 20
  HR : Inport
  Enable : EnablePort
  Add{1..12,19} (13 alike) : Sum
  Constant1 : Constant  Value=800
  Constant2 : Constant  Value=1100
  Constant20 : Constant  Value=20
  Constant3 : Constant  Value=27
  Constant4 : Constant  Value=-20
  Constant5 : Constant  Value=158
  Constant6 : Constant  Value=77
  Gain1 : Gain  Gain=6.6667
  Gain10 : Gain  Gain=4.5
  Gain11 : Gain  Gain=1/100
  Gain12 : Gain  Gain=0.0156
  Gain13 : Gain  Gain=-1.9333
  Gain14 : Gain  Gain=-0.0006
  Gain15 : Gain  Gain=-0.4167
  Gain16 : Gain  Gain=-2e-15
  Gain2 : Gain  Gain=-0.0556
  Gain3 : Gain  Gain=0.8333
  Gain4 : Gain  Gain=-1.6667
  Gain5 : Gain  Gain=1/10
  Gain6 : Gain  Gain=0.005
  Gain7 : Gain  Gain=0.083
  Gain9 : Gain  Gain=-0.0111
  Mux : Mux  Inputs=7
  Product{1..6} (6 alike) : Product
  Scope : Scope
      settings: ActiveDisplayYMinimum=60  ActiveDisplayYMaximum=80  DataLoggingVariableName=ScopeData4
  Scope2 : Scope
      settings: ActiveDisplayYMinimum=0.88246  ActiveDisplayYMaximum=1.08246  DataLoggingVariableName=ScopeData5
  Output : Outport
  wires:
  HR/1 -> Gain3/1, Product5/2, Gain1/1, Product5/1, Gain7/1, Product1/2, Gain10/1, Product2/2, Product2/1, Product4/1, Product4/2, Gain15/1, Product3/1, Product3/2, Gain13/1, Product1/1, Gain4/1, Product6/2, Product6/1
  Add12/1 -> Add2/1
  Add5/1 -> Add6/1
  Gain2/1 -> Add11/1
  Constant20/1 -> Add19/2
  Gain4/1 -> Add12/2
  Add1/1 -> Mux/2
  Add3/1 -> Add4/1
  Add11/1 -> Add1/1
  Add10/1 -> Mux/7
  Gain5/1 -> Mux/4
  Constant5/1 -> Add8/2
  Add19/1 -> Scope/1, Mux/1
  Gain3/1 -> Add19/1
  Gain15/1 -> Add9/2
  Add9/1 -> Add10/1
  Gain14/1 -> Add9/1
  Product3/1 -> Gain12/1
  Constant1/1 -> Add1/2
  Mux/1 -> Output/1
  Constant2/1 -> Add2/2
  Gain6/1 -> Add3/1
  Constant4/1 -> Add6/2
  Product2/1 -> Gain9/1
  Add7/1 -> Add8/1
  Gain7/1 -> Add3/2
  Add8/1 -> Gain11/1
  Product1/1 -> Gain6/1
  Gain11/1 -> Scope2/1, Mux/5
  Gain9/1 -> Add5/1
  Gain10/1 -> Add5/2
  Constant3/1 -> Add4/2
  Add2/1 -> Mux/3
  Gain16/1 -> Add12/1
  Gain12/1 -> Add7/1
  Constant6/1 -> Add10/2
  Gain13/1 -> Add7/2
  Product4/1 -> Gain14/1
  Add4/1 -> Gain5/1
  Gain1/1 -> Add11/2
  Product5/1 -> Gain2/1
  Product6/1 -> Gain16/1
  Add6/1 -> Mux/6

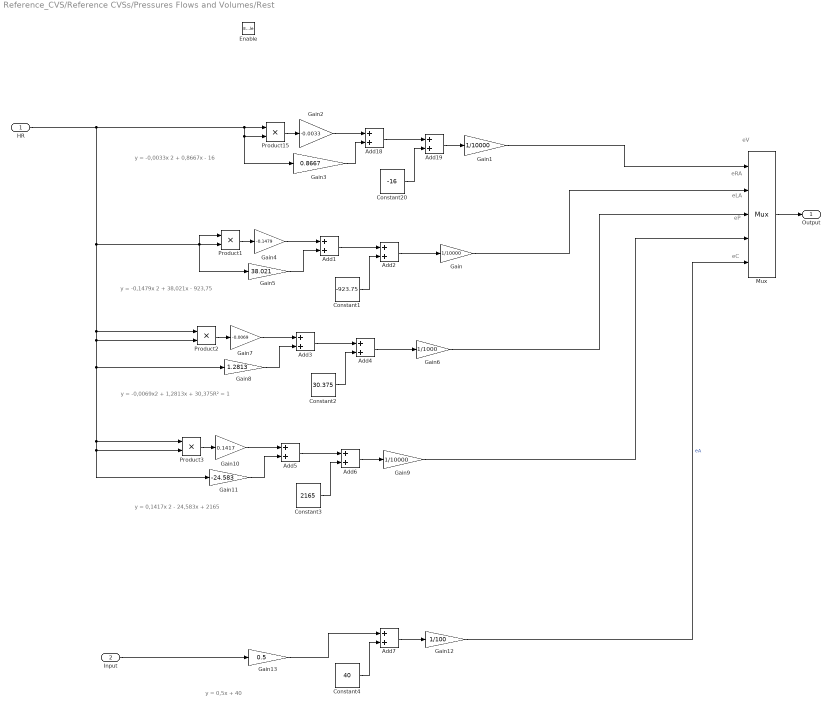
== system Reference_CVS/Reference CVSs/Pressures Flows and Volumes/Rest ==
  note: eV
  note: y = 0,5x + 40
  note: y = -0,1479x 2 + 38,021x - 923,75
  note: y = -0,0069x2 + 1,2813x + 30,375R² = 1
  note: y = 0,1417x 2 - 24,583x + 2165
  note: eP
  note: eLA
  note: eRA
  note: y = -0,0033x 2 + 0,8667x - 16
  note: eC
  HR : Inport
  Input : Inport  Port=2
  Enable : EnablePort
  Add{1..7,18..19} (9 alike) : Sum
  Constant1 : Constant  Value=-923.75
  Constant2 : Constant  Value=30.375
  Constant20 : Constant  Value=-16
  Constant3 : Constant  Value=2165
  Constant4 : Constant  Value=40
  Gain : Gain  Gain=1/10000
  Gain1 : Gain  Gain=1/10000
  Gain10 : Gain  Gain=0.1417
  Gain11 : Gain  Gain=-24.583
  Gain12 : Gain  Gain=1/100
  Gain13 : Gain  Gain=0.5
  Gain2 : Gain  Gain=-0.0033
  Gain3 : Gain  Gain=0.8667
  Gain4 : Gain  Gain=-0.1479
  Gain5 : Gain  Gain=38.021
  Gain6 : Gain  Gain=1/1000
  Gain7 : Gain  Gain=-0.0069
  Gain8 : Gain  Gain=1.2813
  Gain9 : Gain  Gain=1/10000
  Mux : Mux  Inputs=5
  Product{1..3,15} (4 alike) : Product
  Output : Outport
  wires:
  Input/1 -> Gain13/1
  Gain12/1 -> Mux/5  "eA"
  Gain13/1 -> Add7/1
  Constant4/1 -> Add7/2
  Add7/1 -> Gain12/1
  Add6/1 -> Gain9/1
  Gain11/1 -> Add5/2
  Gain10/1 -> Add5/1
  Constant3/1 -> Add6/2
  Product3/1 -> Gain10/1
  Add5/1 -> Add6/1
  HR/1 -> Product15/1, Product15/2, Gain3/1, Gain11/1, Product3/2, Product3/1, Gain8/1, Product2/2, Product2/1, Product1/2, Gain5/1, Product1/1
  Product2/1 -> Gain7/1
  Gain8/1 -> Add3/2
  Add4/1 -> Gain6/1
  Add3/1 -> Add4/1
  Constant2/1 -> Add4/2
  Gain7/1 -> Add3/1
  Product1/1 -> Gain4/1
  Add1/1 -> Add2/1
  Add2/1 -> Gain/1
  Constant1/1 -> Add2/2
  Gain5/1 -> Add1/2
  Gain4/1 -> Add1/1
  Gain9/1 -> Mux/4
  Gain/1 -> Mux/2
  Mux/1 -> Output/1
  Gain6/1 -> Mux/3
  Gain1/1 -> Mux/1
  Add18/1 -> Add19/1
  Gain2/1 -> Add18/1
  Constant20/1 -> Add19/2
  Add19/1 -> Gain1/1
  Product15/1 -> Gain2/1
  Gain3/1 -> Add18/2

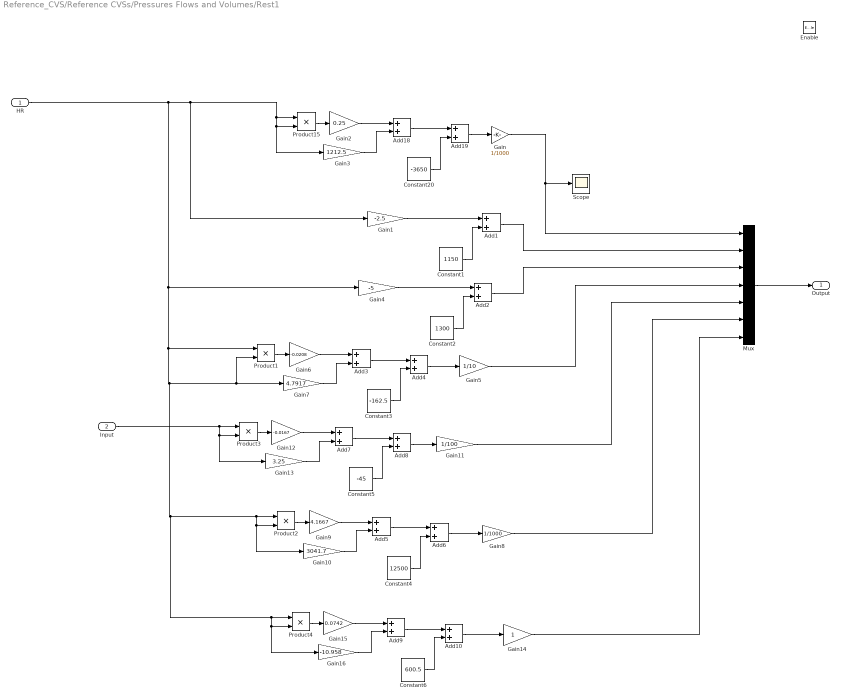
== system Reference_CVS/Reference CVSs/Pressures Flows and Volumes/Rest1 ==
  HR : Inport
  Input : Inport  Port=2
  Enable : EnablePort
  Add{1..10,18..19} (12 alike) : Sum
  Constant1 : Constant  Value=1150
  Constant2 : Constant  Value=1300
  Constant20 : Constant  Value=-3650
  Constant3 : Constant  Value=-162.5
  Constant4 : Constant  Value=12500
  Constant5 : Constant  Value=-45
  Constant6 : Constant  Value=600.5
  Gain : Gain  Gain=1/1000
  Gain1 : Gain  Gain=-2.5
  Gain10 : Gain  Gain=3041.7
  Gain11 : Gain  Gain=1/100
  Gain12 : Gain  Gain=-0.0167
  Gain13 : Gain  Gain=3.25
  Gain14 : Gain
  Gain15 : Gain  Gain=0.0742
  Gain16 : Gain  Gain=-10.958
  Gain2 : Gain  Gain=0.25
  Gain3 : Gain  Gain=1212.5
  Gain4 : Gain  Gain=-5
  Gain5 : Gain  Gain=1/10
  Gain6 : Gain  Gain=-0.0208
  Gain7 : Gain  Gain=4.7917
  Gain8 : Gain  Gain=1/1000
  Gain9 : Gain  Gain=4.1667
  Mux : Mux  Inputs=7
  Product{1..4,15} (5 alike) : Product
  Scope : Scope
      settings: ActiveDisplayYMinimum=60  ActiveDisplayYMaximum=80  DataLoggingVariableName=ScopeData9
  Output : Outport
  wires:
  Gain16/1 -> Add9/2
  Gain14/1 -> Mux/7
  Gain15/1 -> Add9/1
  HR/1 -> Gain3/1, Product15/2, Product15/1, Gain1/1, Gain7/1, Product1/2, Gain10/1, Product2/2, Product2/1, Gain16/1, Product4/2, Product4/1, Product1/1, Gain4/1
  Add10/1 -> Gain14/1
  Constant6/1 -> Add10/2
  Add9/1 -> Add10/1
  Product4/1 -> Gain15/1
  Gain11/1 -> Mux/5
  Input/1 -> Gain13/1, Product3/2, Product3/1
  Gain12/1 -> Add7/1
  Add8/1 -> Gain11/1
  Constant5/1 -> Add8/2
  Product3/1 -> Gain12/1
  Add7/1 -> Add8/1
  Gain13/1 -> Add7/2
  Gain9/1 -> Add5/1
  Product2/1 -> Gain9/1
  Add5/1 -> Add6/1
  Gain8/1 -> Mux/6
  Gain10/1 -> Add5/2
  Constant4/1 -> Add6/2
  Add6/1 -> Gain8/1
  Add3/1 -> Add4/1
  Add4/1 -> Gain5/1
  Gain6/1 -> Add3/1
  Product1/1 -> Gain6/1
  Gain5/1 -> Mux/4
  Gain7/1 -> Add3/2
  Constant3/1 -> Add4/2
  Constant2/1 -> Add2/2
  Add2/1 -> Mux/3
  Gain4/1 -> Add2/1
  Gain1/1 -> Add1/1
  Constant1/1 -> Add1/2
  Add1/1 -> Mux/2
  Add18/1 -> Add19/1
  Add19/1 -> Gain/1
  Gain3/1 -> Add18/2
  Product15/1 -> Gain2/1
  Constant20/1 -> Add19/2
  Gain/1 -> Scope/1, Mux/1
  Gain2/1 -> Add18/1
  Mux/1 -> Output/1

== system Reference_CVS/Reference CVSs/Pressures Flows and Volumes/Subsystem13 ==
  note: y = 0,1944x 2 - 28,333x + 1100
  note: y = 0,0083x 2 - 0,9167x + 40
  Add{1..2,18..19} (4 alike) : Sum
  Constant1 : Constant  Value=40
  Constant20 : Constant  Value=1100
  Display : Display
  Gain : Gain  Gain=1/10
  Gain2 : Gain  Gain=0.1944
  Gain3 : Gain  Gain=-28.333
  Gain4 : Gain  Gain=0.0083
  Gain5 : Gain  Gain=-0.9167
  Product1 : Product
  Product15 : Product
  Scope : Scope
      settings: ActiveDisplayYMinimum=8.99968  ActiveDisplayYMaximum=10.99968  DataLoggingVariableName=ScopeData2
  Scope1 : Scope
      settings: ActiveDisplayYMinimum=8.99968  ActiveDisplayYMaximum=10.99968
  Switch : Switch  Criteria=u2 > Threshold  SaturateOnIntegerOverflow=off  InputSameDT=off
  V0 : Outport
  wires:
  Switch/1 -> V0/1, Display/1
  [Heart_Failure_On_Off] -> Switch/2
  Add1/1 -> Add2/1
  Gain5/1 -> Add1/2
  Product1/1 -> Gain4/1
  Constant1/1 -> Add2/2
  Gain4/1 -> Add1/1
  [HR] -> Product1/1, Product1/2, Gain5/1
  Add2/1 -> Scope1/1, Switch/1
  Gain/1 -> Scope/1, Switch/3
  [HR] -> Gain3/1, Product15/2, Product15/1
  Gain2/1 -> Add18/1
  Constant20/1 -> Add19/2
  Product15/1 -> Gain2/1
  Gain3/1 -> Add18/2
  Add18/1 -> Add19/1
  Add19/1 -> Gain/1

== system Reference_CVS/Reference CVSs/Pressures Flows and Volumes/Subsystem5 ==
  In1 : Inport
  elv : Inport  Port=2
  erv : Inport  Port=3
  In4 : Inport  Port=4
  Switch : Switch  Criteria=u2 > Threshold  SaturateOnIntegerOverflow=off  InputSameDT=off
  Switch4 : Switch  Criteria=u2 > Threshold  SaturateOnIntegerOverflow=off  InputSameDT=off
  VolumesForVAD : Subsystem
  Out1 : Outport
  Output1 : Outport  Port=2
  wires:
  In4/1 -> Switch4/3
  Switch/1 -> Out1/1
  Switch4/1 -> Output1/1
  In1/1 -> Switch/3
  VolumesForVAD/1(Output2) -> Switch/1
  erv/1 -> VolumesForVAD/2(erv1)
  VolumesForVAD/2(Output1) -> Switch4/1
  elv/1 -> VolumesForVAD/1(elv1)
  [QVAD] -> Switch/2, Switch4/2

== system Reference_CVS/Reference CVSs/eLV/LV_e_min ==
  VLV : Inport
  Add : Sum  Inputs=+-
  Add1 : Sum  Inputs=+-
  Add2 : Sum
  Constant9 : Constant
  Display : Display
  Display1 : Display
  Exp : Math  SignedPower=on
  Product : Product
  Product1 : Product
  Real_CLV : Subsystem
  Subsystem1 : Subsystem
  Subsystem2 : Subsystem
  Subsystem5 : Subsystem
  Switch : Switch  Criteria=u2 > Threshold  SaturateOnIntegerOverflow=off  InputSameDT=off
  Switch1 : Switch  Criteria=u2 > Threshold  SaturateOnIntegerOverflow=off  InputSameDT=off
  Switch2 : Switch  Criteria=u2 > Threshold  SaturateOnIntegerOverflow=off  InputSameDT=off
  a_LV_Cons : Constant  Value=0.4641
  d_LV_Cons : Constant  Value=0.1235
  resting : Subsystem
  eLV_min_O : Outport
  tag scope: bLV=global, cLV=global
  wires:
  Switch1/1 -> Display1/1, Add/2, [cLV]
  Switch2/1 -> Switch/3
  Switch/1 -> Display/1, Product1/1, [bLV]
  Subsystem2/1(B_LV) -> Switch2/1
  resting/1(B_LV) -> Switch2/3
  [Exercise_On_Off] -> Switch2/2
  Subsystem5/1(B_LV_HF) -> Switch/1
  Real_CLV/1(C_LV) -> Switch1/1
  [Heart_Failure_On_Off] -> Switch1/2
  Subsystem1/1(C_LV) -> Switch1/3
  [Heart_Failure_On_Off] -> Switch/2
  a_LV_Cons/1 -> Product/1
  Add2/1 -> eLV_min_O/1
  VLV/1 -> Add/1
  Constant9/1 -> Add1/2
  Add1/1 -> Product/2
  Product/1 -> Add2/1
  d_LV_Cons/1 -> Add2/2
  Exp/1 -> Add1/1
  Product1/1 -> Exp/1
  Add/1 -> Product1/2

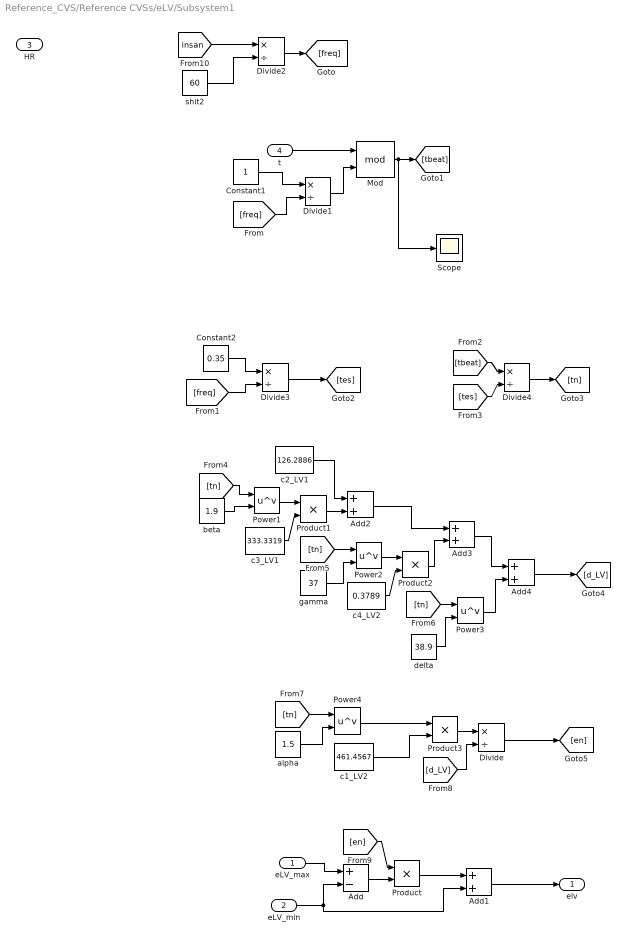
== system Reference_CVS/Reference CVSs/eLV/Subsystem1 ==
  eLV_max : Inport
  eLV_min : Inport  Port=2
  HR : Inport  Port=3
  t : Inport  Port=4
  Add : Sum  Inputs=+-
  Add{1..4} (4 alike) : Sum
  Constant1 : Constant
  Constant2 : Constant  Value=0.35
  Divide{,1..4} (5 alike) : Product  Inputs=*/  RndMeth=Zero  SaturateOnIntegerOverflow=on
  Mod : Math  Operator=mod  SignedPower=on
  Power{1..4} (4 alike) : Math  Operator=pow  SignedPower=on
  Product{,1..3} (4 alike) : Product
  Scope : Scope
      settings: ActiveDisplayYMinimum=-0.05357  ActiveDisplayYMaximum=0.43719  DataLoggingVariableName=ScopeData4
  alpha : Constant  Value=1.5
  beta : Constant  Value=1.9
  c1_LV2 : Constant  Value=461.4567
  c2_LV1 : Constant  Value=126.2886
  c3_LV1 : Constant  Value=333.3319
  c4_LV2 : Constant  Value=0.3789
  delta : Constant  Value=38.9
  gamma : Constant  Value=37
  "shit2 " : Constant  Value=60
  elv : Outport
  wires:
  [insan] -> Divide2/1
  Mod/1 -> [tbeat], Scope/1
  Divide1/1 -> Mod/2
  t/1 -> Mod/1
  [en] -> Product/1
  [d_LV] -> Divide/2
  Divide/1 -> [en]
  Product3/1 -> Divide/1
  c1_LV2/1 -> Product3/2
  Power4/1 -> Product3/1
  alpha/1 -> Power4/2
  [tn] -> Power4/1
  Add4/1 -> [d_LV]
  Power3/1 -> Add4/2
  Add3/1 -> Add4/1
  delta/1 -> Power3/2
  [tn] -> Power3/1
  Product2/1 -> Add3/2
  c4_LV2/1 -> Product2/2
  Power2/1 -> Product2/1
  gamma/1 -> Power2/2
  [tn] -> Power2/1
  Add2/1 -> Add3/1
  Product1/1 -> Add2/2
  c3_LV1/1 -> Product1/2
  Power1/1 -> Product1/1
  beta/1 -> Power1/2
  [tn] -> Power1/1
  c2_LV1/1 -> Add2/1
  Divide4/1 -> [tn]
  [tes] -> Divide4/2
  [tbeat] -> Divide4/1
  Divide3/1 -> [tes]
  [freq] -> Divide3/2
  Constant2/1 -> Divide3/1
  Constant1/1 -> Divide1/1
  [freq] -> Divide1/2
  Divide2/1 -> [freq]
  "shit2 "/1 -> Divide2/2
  eLV_max/1 -> Add/1
  eLV_min/1 -> Add1/2, Add/2
  Add1/1 -> elv/1
  Add/1 -> Product/2
  Product/1 -> Add1/1

== system Reference_CVS/Reference CVSs/eLV/eLV1 ==
  note: y = 0,0027x 2 - 0,0767x + 24,76
  Add18 : Sum
  Add19 : Sum
  Constant20 : Constant  Value=24.76
  Gain1 : Gain  Gain=1/10
  Gain2 : Gain  Gain=0.0027
  Gain3 : Gain  Gain=-0.0767
  PID : Subsystem  Commented=on
  Product15 : Product
  Scope : Scope
      settings: ActiveDisplayYMinimum=2.20237  ActiveDisplayYMaximum=2.60692
  Stair Generator : powerlib_meascontrol/Pulse & Signal Generators/Stair Generator  Commented=on  t=[0,50,100,150]  e=[3.25,3.5,3.75,4]  Ts=stepsize
      settings: SourceProductName=Simscape Electrical
  Stair Generator1 : powerlib_meascontrol/Pulse & Signal Generators/Stair Generator  Commented=on  t=[100,200,300,400]  e=[3.25,3.5,3.75,4]  Ts=stepsize
      settings: SourceProductName=Simscape Electrical
  Output : Outport
  wires:
  Gain1/1 -> Output/1, Scope/1
  Constant20/1 -> Add19/2
  Product15/1 -> Gain2/1
  Add18/1 -> Add19/1
  [HR] -> Gain3/1, Product15/2, Product15/1
  Gain3/1 -> Add18/2
  Gain2/1 -> Add18/1
  Add19/1 -> Gain1/1
  Stair Generator1/1 -> PID/1(s)

== system Reference_CVS/Reference CVSs/eLV/eLVsick ==
  note: y = -0,0028x 2 + 0,9167x + 45
  Add18 : Sum
  Add19 : Sum
  Constant20 : Constant  Value=45
  Gain1 : Gain  Gain=1/100
  Gain2 : Gain  Gain=-0.0028
  Gain3 : Gain  Gain=0.9167
  Product15 : Product
  Scope : Scope
      settings: ActiveDisplayYMinimum=2.20237  ActiveDisplayYMaximum=2.60692  DataLoggingVariableName=ScopeData6
  Output : Outport
  wires:
  Add19/1 -> Gain1/1
  Add18/1 -> Add19/1
  [HR] -> Gain3/1, Product15/2, Product15/1
  Gain2/1 -> Add18/1
  Constant20/1 -> Add19/2
  Gain3/1 -> Add18/2
  Gain1/1 -> Output/1, Scope/1
  Product15/1 -> Gain2/1

== system Reference_CVS/Reference CVSs/eRV/RV_e_min ==
  VRV : Inport
  Add3 : Sum  Inputs=+-
  Add4 : Sum
  Constant13 : Constant
  Display1 : Display
  Exp1 : Math  SignedPower=on
  Product2 : Product
  Product3 : Product
  Switch1 : Switch  Criteria=u2 > Threshold  Threshold=0.9  SaturateOnIntegerOverflow=off  InputSameDT=off
  a_RV_Cons : Constant  Value=0.03752
  b_RV_Cons : Constant  Value=0.03776
  c_RV : Subsystem
  real_c_RV : Subsystem
  eRV_min_O : Outport
  tag scope: cRV=global
  wires:
  c_RV/1(Output) -> Switch1/3
  [Heart_Failure_On_Off] -> Switch1/2
  real_c_RV/1(Output) -> Switch1/1
  Product3/1 -> eRV_min_O/1
  b_RV_Cons/1 -> Product2/2
  a_RV_Cons/1 -> Product3/1
  Switch1/1 -> [cRV], Add3/2, Display1/1
  Add4/1 -> Product3/2
  Exp1/1 -> Add4/1
  VRV/1 -> Add3/1
  Add3/1 -> Product2/1
  Product2/1 -> Exp1/1
  Constant13/1 -> Add4/2

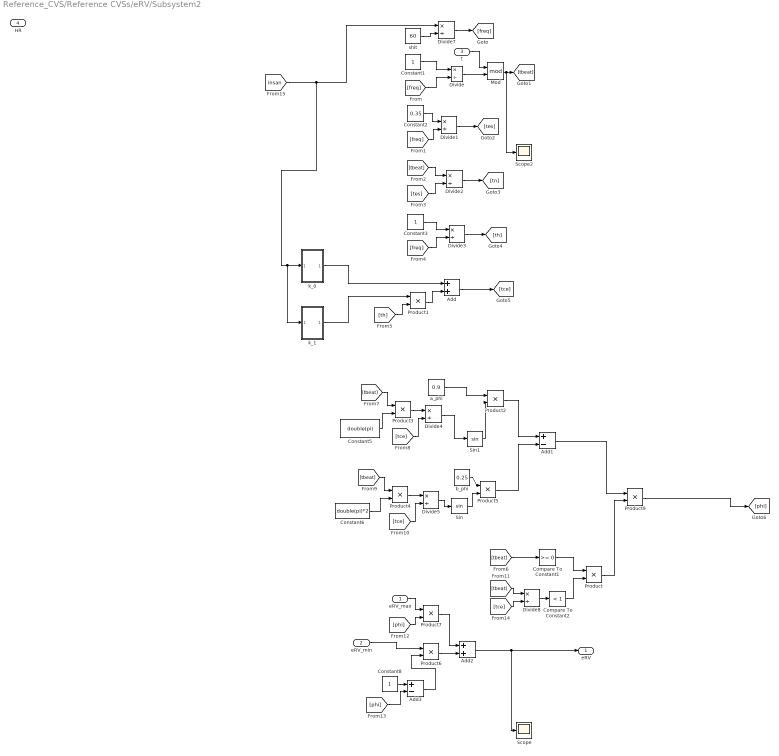
== system Reference_CVS/Reference CVSs/eRV/Subsystem2 ==
  eRV_max : Inport
  eRV_min : Inport  Port=2
  t : Inport  Port=3
  HR : Inport  Port=4
  Add : Sum
  Add1 : Sum  Inputs=+-
  Add2 : Sum
  Add3 : Sum  Inputs=+-
  Compare To Constant1 : simulink/Logic and Bit Operations/Compare To Constant  relop=>=  const=0  OutDataTypeStr=boolean
  Compare To Constant2 : simulink/Logic and Bit Operations/Compare To Constant  relop=<  const=1  OutDataTypeStr=boolean
  Constant1 : Constant
  Constant2 : Constant  Value=0.35
  Constant3 : Constant
  Constant5 : Constant  Value=double(pi)
  Constant6 : Constant  Value=double(pi)*2
  Constant8 : Constant
  Divide{,1..5,7..8} (8 alike) : Product  Inputs=*/  RndMeth=Zero  SaturateOnIntegerOverflow=on
  Mod : Math  Operator=mod  SignedPower=on
  Product{,1..7,9} (9 alike) : Product
  Scope : Scope
      settings: ActiveDisplayYMinimum=-0.03117  ActiveDisplayYMaximum=2.17237  DataLoggingVariableName=ScopeData3
  Scope2 : Scope
      settings: ActiveDisplayYMinimum=-0.09374  ActiveDisplayYMaximum=0.84364  DataLoggingVariableName=ScopeData6
  Sin : Trigonometry
  Sin1 : Trigonometry
  a_phi : Constant  Value=0.9
  b_phi : Constant  Value=0.25
  k_0 : Subsystem
  k_1 : Subsystem
  shit : Constant  Value=60
  eRV : Outport
  wires:
  [insan] -> Divide7/1, k_0/1(In1), k_1/1(In1)
  k_0/1(Out1) -> Add/1
  k_1/1(Out1) -> Product1/1
  Sin1/1 -> Product2/2
  Divide4/1 -> Sin1/1
  Product/1 -> Product9/2
  Compare To Constant2/1 -> Product/2
  Compare To Constant1/1 -> Product/1
  Divide8/1 -> Compare To Constant2/1
  [tce] -> Divide8/2
  [tbeat] -> Divide8/1
  t/1 -> Mod/1
  Divide/1 -> Mod/2
  Add3/1 -> Product6/2
  [phi] -> Add3/2
  Constant8/1 -> Add3/1
  Add2/1 -> eRV/1, Scope/1
  Product7/1 -> Add2/1
  [phi] -> Product7/2
  eRV_max/1 -> Product7/1
  Product6/1 -> Add2/2
  eRV_min/1 -> Product6/1
  Product9/1 -> [phi]
  Add1/1 -> Product9/1
  Product5/1 -> Add1/2
  b_phi/1 -> Product5/1
  Sin/1 -> Product5/2
  Product4/1 -> Divide5/1
  [tbeat] -> Product4/1
  [tce] -> Divide5/2
  Constant6/1 -> Product4/2
  Divide5/1 -> Sin/1
  Product2/1 -> Add1/1
  [tce] -> Divide4/2
  Product3/1 -> Divide4/1
  Constant5/1 -> Product3/2
  [tbeat] -> Product3/1
  a_phi/1 -> Product2/1
  [tbeat] -> Compare To Constant1/1
  Product1/1 -> Add/2
  Add/1 -> [tce]
  [th] -> Product1/2
  Divide3/1 -> [th]
  [freq] -> Divide3/2
  Constant3/1 -> Divide3/1
  Divide2/1 -> [tn]
  [tes] -> Divide2/2
  [tbeat] -> Divide2/1
  Divide1/1 -> [tes]
  [freq] -> Divide1/2
  Constant2/1 -> Divide1/1
  Mod/1 -> [tbeat], Scope2/1
  [freq] -> Divide/2
  Constant1/1 -> Divide/1
  Divide7/1 -> [freq]
  shit/1 -> Divide7/2

== system Reference_CVS/Reference CVSs/eRV/eRV2 ==
  note: y = 0,005x 2 + 0,25x + 17
  Add18 : Sum
  Add19 : Sum
  Constant20 : Constant  Value=17
  Gain1 : Gain  Gain=1/100
  Gain2 : Gain  Gain=0.005
  Gain3 : Gain  Gain=0.25
  PID : Subsystem  Commented=on
  Product15 : Product
  Scope : Scope
      settings: ActiveDisplayYMinimum=1.07059  ActiveDisplayYMaximum=1.42514
  Stair Generator : powerlib_meascontrol/Pulse & Signal Generators/Stair Generator  Commented=on  t=[0,50,100,150]  e=[3.25,3.5,3.75,4]  Ts=stepsize
      settings: SourceProductName=Simscape Electrical
  Stair Generator1 : powerlib_meascontrol/Pulse & Signal Generators/Stair Generator  Commented=on  t=[100,200,300,400]  e=[3.25,3.5,3.75,4]  Ts=stepsize
      settings: SourceProductName=Simscape Electrical
  Output : Outport
  wires:
  Stair Generator1/1 -> PID/1(s)
  Add19/1 -> Gain1/1
  Gain2/1 -> Add18/1
  Gain3/1 -> Add18/2
  [HR] -> Product15/1, Product15/2, Gain3/1
  Add18/1 -> Add19/1
  Product15/1 -> Gain2/1
  Constant20/1 -> Add19/2
  Gain1/1 -> Scope/1, Output/1

== system Reference_CVS/Reference CVSs/eRV/eRVhf ==
  note: y = 0,0056x 2 - 0,6667x + 60
  Add18 : Sum
  Add19 : Sum
  Constant20 : Constant  Value=60
  Gain1 : Gain  Gain=1/100
  Gain2 : Gain  Gain=0.0056
  Gain3 : Gain  Gain=-0.6667
  PID : Subsystem  Commented=on
  Product15 : Product
  Scope : Scope
      settings: ActiveDisplayYMinimum=1.07059  ActiveDisplayYMaximum=1.42514
  Stair Generator : powerlib_meascontrol/Pulse & Signal Generators/Stair Generator  Commented=on  t=[0,50,100,150]  e=[3.25,3.5,3.75,4]  Ts=stepsize
      settings: SourceProductName=Simscape Electrical
  Stair Generator1 : powerlib_meascontrol/Pulse & Signal Generators/Stair Generator  Commented=on  t=[100,200,300,400]  e=[3.25,3.5,3.75,4]  Ts=stepsize
      settings: SourceProductName=Simscape Electrical
  Output : Outport
  wires:
  Stair Generator1/1 -> PID/1(s)
  Add19/1 -> Gain1/1
  Gain2/1 -> Add18/1
  Gain3/1 -> Add18/2
  [HR] -> Product15/1, Product15/2, Gain3/1
  Add18/1 -> Add19/1
  Product15/1 -> Gain2/1
  Constant20/1 -> Add19/2
  Gain1/1 -> Scope/1, Output/1
